simulink library "MathLibrary"  (R2017b)
settings: Solver=VariableStepAuto  StartTime=0.0  StopTime=10.0  RelTol=1e-3
undefined symbols (not defined in the file): magnitude
settings Model: Creator=Holzapfel  LastModifiedBy=zht
settings CodeAppCC: StateflowObjectComments=on

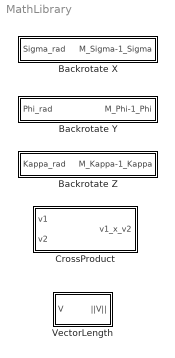
== system MathLibrary ==
  Backrotate X : Subsystem
  Backrotate Y : Subsystem
  Backrotate Z : Subsystem
  CrossProduct : Subsystem
  VectorLength : Subsystem

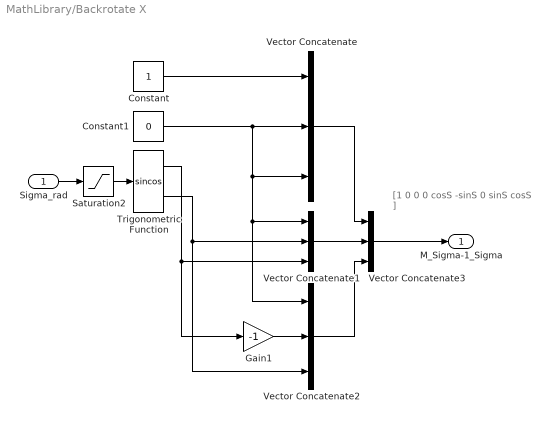
== system MathLibrary/Backrotate X ==
  note: [1        0           0
      |  0        cosS     -sinS
      |  0        sinS      cosS ]
  Sigma_rad : Inport  Unit=rad  PortDimensions=[1,1]
  Constant : Constant
  Constant1 : Constant  Value=0
  Gain1 : Gain  Gain=-1
  Saturation2 : Saturate  UpperLimit=pi  LowerLimit=-pi
  Trigonometric Function : Trigonometry  Operator=sincos  NumberOfIterations=15
  Vector Concatenate : Concatenate  NumInputs=3
  Vector Concatenate1 : Concatenate  NumInputs=3
  Vector Concatenate2 : Concatenate  NumInputs=3
  Vector Concatenate3 : Concatenate  NumInputs=3  Mode=Multidimensional array  ConcatenateDimension=2
  M_Sigma-1_Sigma : Outport  PortDimensions=[3,3]
  wires:
  Vector Concatenate3/1 -> M_Sigma-1_Sigma/1
  Vector Concatenate2/1 -> Vector Concatenate3/3
  Vector Concatenate1/1 -> Vector Concatenate3/2
  Vector Concatenate/1 -> Vector Concatenate3/1
  Sigma_rad/1 -> Saturation2/1
  Constant/1 -> Vector Concatenate/1
  Constant1/1 -> Vector Concatenate2/1, Vector Concatenate1/1, Vector Concatenate/3, Vector Concatenate/2
  Trigonometric Function/2 -> Vector Concatenate2/3, Vector Concatenate1/2
  Trigonometric Function/1 -> Gain1/1, Vector Concatenate1/3
  Gain1/1 -> Vector Concatenate2/2
  Saturation2/1 -> Trigonometric Function/1

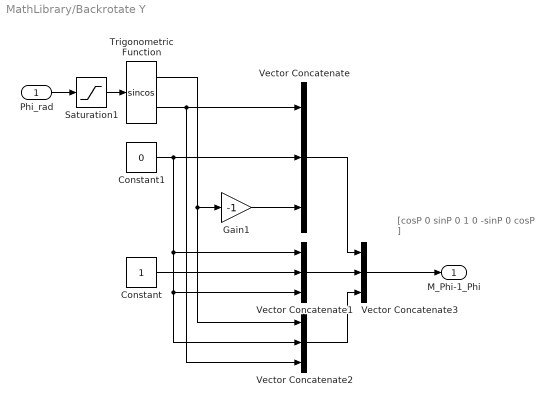
== system MathLibrary/Backrotate Y ==
  note: [cosP  0     sinP
      |  0        1     0
      | -sinP   0     cosP ]
  Phi_rad : Inport  Unit=rad  PortDimensions=[1,1]
  Constant : Constant
  Constant1 : Constant  Value=0
  Gain1 : Gain  Gain=-1
  Saturation1 : Saturate  UpperLimit=4*pi  LowerLimit=-4*pi
  Trigonometric Function : Trigonometry  Operator=sincos  NumberOfIterations=15
  Vector Concatenate : Concatenate  NumInputs=3
  Vector Concatenate1 : Concatenate  NumInputs=3
  Vector Concatenate2 : Concatenate  NumInputs=3
  Vector Concatenate3 : Concatenate  NumInputs=3  Mode=Multidimensional array  ConcatenateDimension=2
  M_Phi-1_Phi : Outport  PortDimensions=[3,3]
  wires:
  Phi_rad/1 -> Saturation1/1
  Trigonometric Function/2 -> Vector Concatenate2/3, Vector Concatenate/1
  Constant1/1 -> Vector Concatenate2/2, Vector Concatenate1/3, Vector Concatenate1/1, Vector Concatenate/2
  Trigonometric Function/1 -> Vector Concatenate2/1, Gain1/1
  Gain1/1 -> Vector Concatenate/3
  Vector Concatenate/1 -> Vector Concatenate3/1
  Vector Concatenate1/1 -> Vector Concatenate3/2
  Vector Concatenate2/1 -> Vector Concatenate3/3
  Constant/1 -> Vector Concatenate1/2
  Vector Concatenate3/1 -> M_Phi-1_Phi/1
  Saturation1/1 -> Trigonometric Function/1

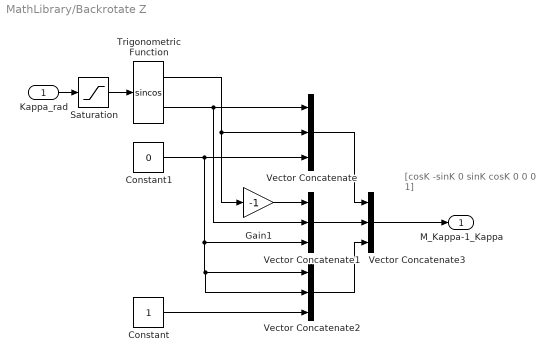
== system MathLibrary/Backrotate Z ==
  note: [cosK -sinK    0
      |  sinK   cosK   0
      |  0         0        1]
  Kappa_rad : Inport  Unit=rad  PortDimensions=[1,1]
  Constant : Constant
  Constant1 : Constant  Value=0
  Gain1 : Gain  Gain=-1
  Saturation : Saturate  UpperLimit=375*pi/180  LowerLimit=-375*pi/180
  Trigonometric Function : Trigonometry  Operator=sincos  NumberOfIterations=15
  Vector Concatenate : Concatenate  NumInputs=3
  Vector Concatenate1 : Concatenate  NumInputs=3
  Vector Concatenate2 : Concatenate  NumInputs=3
  Vector Concatenate3 : Concatenate  NumInputs=3  Mode=Multidimensional array  ConcatenateDimension=2
  M_Kappa-1_Kappa : Outport  PortDimensions=[3,3]
  wires:
  Kappa_rad/1 -> Saturation/1
  Vector Concatenate/1 -> Vector Concatenate3/1
  Vector Concatenate1/1 -> Vector Concatenate3/2
  Vector Concatenate2/1 -> Vector Concatenate3/3
  Vector Concatenate3/1 -> M_Kappa-1_Kappa/1
  Trigonometric Function/2 -> Vector Concatenate1/2, Vector Concatenate/1
  Trigonometric Function/1 -> Gain1/1, Vector Concatenate/2
  Constant1/1 -> Vector Concatenate2/2, Vector Concatenate2/1, Vector Concatenate1/3, Vector Concatenate/3
  Gain1/1 -> Vector Concatenate1/1
  Constant/1 -> Vector Concatenate2/3
  Saturation/1 -> Trigonometric Function/1

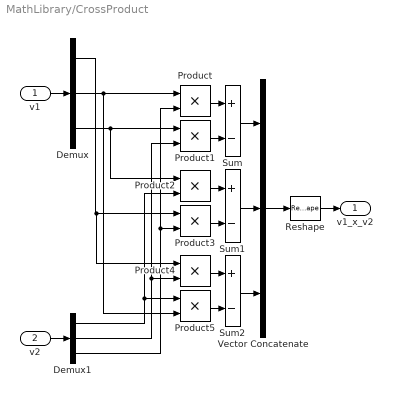
== system MathLibrary/CrossProduct ==
  v1 : Inport  PortDimensions=[3,1]
  v2 : Inport  Port=2  PortDimensions=[3,1]
  Demux : Demux  Outputs=3
  Demux1 : Demux  Outputs=3
  Product{,1..5} (6 alike) : Product
  Reshape : Reshape  OutputDimensionality=Column vector (2-D)  OutputDimensions=1
  Sum : Sum  Inputs=+-
  Sum1 : Sum  Inputs=+-
  Sum2 : Sum  Inputs=+-
  Vector Concatenate : Concatenate  NumInputs=3
  v1_x_v2 : Outport  PortDimensions=[3,1]
  wires:
  v1/1 -> Demux/1
  v2/1 -> Demux1/1
  Vector Concatenate/1 -> Reshape/1
  Reshape/1 -> v1_x_v2/1
  Demux/2 -> Product5/2, Product/1
  Demux1/3 -> Product3/2, Product/2
  Demux/3 -> Product1/1, Product2/1
  Demux1/2 -> Product4/2, Product1/2
  Product/1 -> Sum/1
  Product1/1 -> Sum/2
  Product2/1 -> Sum1/1
  Product3/1 -> Sum1/2
  Product4/1 -> Sum2/1
  Product5/1 -> Sum2/2
  Sum/1 -> Vector Concatenate/1
  Sum1/1 -> Vector Concatenate/2
  Sum2/1 -> Vector Concatenate/3
  Demux1/1 -> Product5/1, Product2/2
  Demux/1 -> Product4/1, Product3/1

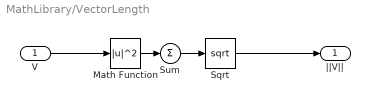
== system MathLibrary/VectorLength ==
  V : Inport
  Math Function : Math  Operator=magnitude^2  SaturateOnIntegerOverflow=on
  Sqrt : Sqrt  SaturateOnIntegerOverflow=on
  Sum : Sum  Inputs=+
  ||V|| : Outport
  wires:
  Math Function/1 -> Sum/1
  Sqrt/1 -> ||V||/1
  Sum/1 -> Sqrt/1
  V/1 -> Math Function/1
